simulink model "EcoSIM3_P2_C2"  (R2014b)
settings: Solver=ode1  SolverMode=SingleTasking  StartTime=0.0  StopTime=inf  FixedStep=0.01  RelTol=1e-3
PostLoadFcn:
  | %, if any(exist('dsrtsu_mdlpostloadfcn', 'file') == [2, 3, 6]), try dsrtsu_mdlpostloadfcn('Execute', bdroot); catch fprintf('Error in PostLoadFcn (dsrtsu_mdlpostloadfcn) for model "%s":\n %s\n', bdroot, lasterr); end, end,
InitFcn:
  | tic
  | %Startup_EcoSIM
undefined symbols (not defined in the file or in its folder): canChannel, Controls, DriveCycles, Driver, EM_EFF_MAP, EM_PwrLoss_MAP, EngPwr, EngSpd, EngTrq, Glbl, Plants, Power, Torque, Veh_Dynamics
libraries: canmsglib x100, canlib x87, fl_lib x78, simulink x59, nesl_utility x40, sdl_lib x17, dspsigops x5, dspswit3 x3, dspstat3 x2, commnoisgen2 x1, dspfdesign x1
(part 4 of 15)

== system EcoSIM3_P2_C2/Powertrain/Accessories/The Corrupter/Switch Logic1 ==
  F : Inport
  L : Inport  Port=2
  NF : Inport  Port=3
  Switch : Switch  Criteria=u2 ~= 0
  Out1 : Outport
  wires:
  L/1 -> Switch/2
  Switch/1 -> Out1/1
  NF/1 -> Switch/3
  F/1 -> Switch/1

== system EcoSIM3_P2_C2/Powertrain/BAS Motor/ Compnent Model/Actuators ==
  note: Actuator Model or a Signal Pass-through, Remove the bus if you are passing through all the signals
  ActuatorInputs : Inport
  Actuator Outputs : Outport
  wires:
  ActuatorInputs/1 -> Actuator Outputs/1

== system EcoSIM3_P2_C2/Powertrain/BAS Motor/ Compnent Model/Plant ==
  note: Component Level Performance Maps
  note: Three kinds of Outputs:
      | 1.To_sensors: Signals that can actually be sensed through Sensors go to sensor models
      | 2. To_plants: Signals that are not actually sensed by sensors but are utilized by the rest of the plant and actually happen physically
      | Component_Logging: Logs both the signal kinds before going through sensor
  note: Motor Speed
  From_Actuators : Inport
  Sensor_Feedback : Inport  Port=2
  BAS Max Torque Curve : Lookup  InputValues=Plants.BAS.Mdl.Plant.max_min_w  Table=Plants.BAS.Mdl.Plant.T_max_Peak  LookUpMeth=Interpolation-Use End Values  SaturateOnIntegerOverflow=on
  BAS Min Torque Curve : Lookup  InputValues=Plants.BAS.Mdl.Plant.max_min_w  Table=Plants.BAS.Mdl.Plant.T_min_Peak  LookUpMeth=Interpolation-Use End Values  SaturateOnIntegerOverflow=on
  Bus Selector : BusSelector  OutputSignals=BAS_Torque_Command_Nm
  Bus Selector1 : BusSelector  OutputSignals=BAS_Speed_rad_per_s
  Ideal Torque Source : fl_lib/Mechanical/Mechanical Sources/Ideal Torque Source
  Inertia : fl_lib/Mechanical/Rotational Elements/Inertia  inertia=0.02 kg*m^2  w_specify=off  w_priority=High  w=0 rad/s  t_specify=off  t_priority=High  t=0 N*m
  Mechanical Rotational Reference : fl_lib/Mechanical/Rotational Elements/Mechanical Rotational Reference
  Saturation Dynamic1 : simulink/Discontinuities/Saturation Dynamic  OutMin=[]  OutMax=[]  OutDataTypeStr=Inherit: Same as second input  OutDataType=sfix(16)  OutScaling=2^-10  DoSatur=off
  Simulink-PS Converter : nesl_utility/Simulink-PS Converter  PhysicalDomain=network_engine_domain  SubClassName=ps_input  LeftPortType=input  RightPortType=output  PseudoPeriodic=off  Frequencies=[]  NoiseDistribution=none  NoiseParameters=[]  Unit=N*m  AffineConversion=off  InputFiltering=off  SimscapeFilterOrder=1  InputFilterTimeConstant=0.001  UdotUserProvided=1
  To_Sensors : PMIOPort  Port=1  Side=Right
  wires:
  From_Actuators/1 -> Bus Selector/1
  BAS Max Torque Curve/1 -> Saturation Dynamic1/1
  BAS Min Torque Curve/1 -> Saturation Dynamic1/3
  Bus Selector/1 -> Saturation Dynamic1/2  "<BAS_Torque_Command_Nm>"
  Saturation Dynamic1/1 -> Simulink-PS Converter/1  "BAS_Torque_Out_Nm"
  Bus Selector1/1 -> BAS Min Torque Curve/1, BAS Max Torque Curve/1  "<BAS_Speed_rad_per_s>"
  Sensor_Feedback/1 -> Bus Selector1/1
  connections:
  Mechanical Rotational Reference/LConn1 -- Ideal Torque Source/RConn2
  Ideal Torque Source/RConn1 -- Simulink-PS Converter/RConn1
  Ideal Torque Source/LConn1 -- Inertia/LConn1 -- To_Sensors/RConn1

== system EcoSIM3_P2_C2/Powertrain/BAS Motor/ Compnent Model/Sensors ==
  note: Sensor Model: Place where we add Corrupter
  Bus Creator : BusCreator  Inputs=3
  Ideal Rotational Motion Sensor : fl_lib/Mechanical/Mechanical Sensors/Ideal Rotational Motion Sensor  offset=0 rad
  Ideal Torque Sensor : fl_lib/Mechanical/Mechanical Sensors/Ideal Torque Sensor
  Mechanical Rotational Reference1 : fl_lib/Mechanical/Rotational Elements/Mechanical Rotational Reference
  PS-Simulink Converter : nesl_utility/PS-Simulink Converter  PhysicalDomain=network_engine_domain  SubClassName=ps_output  LeftPortType=input  RightPortType=output  PseudoPeriodic=off  Frequencies=[]  Unit=rad/s  AffineConversion=off
  PS-Simulink Converter1 : nesl_utility/PS-Simulink Converter  PhysicalDomain=network_engine_domain  SubClassName=ps_output  LeftPortType=input  RightPortType=output  PseudoPeriodic=off  Frequencies=[]  Unit=N*m  AffineConversion=off
  Product : Product
  Sensor lag : Subsystem
  Sensor lag1 : Subsystem
  Shaft : PMIOPort  Port=1  Side=Left
  To_Belt : PMIOPort  Port=2  Side=Right
  Sensor Out : Outport
  Battery : Outport  Port=2
  wires:
  Bus Creator/1 -> Sensor Out/1  "BAS_Sensor_Out"
  Sensor lag/1(o) -> Product/1, Bus Creator/1  "BAS_Speed_rad_per_s"
  PS-Simulink Converter1/1 -> Sensor lag1/1(i)  "BAS_Torque_Out_Nm"
  Product/1 -> Battery/1, Bus Creator/3  "BAS_Power_Out_W"
  PS-Simulink Converter/1 -> Sensor lag/1(i)  "BAS_Speed_rad_per_s"
  Sensor lag1/1(o) -> Product/2, Bus Creator/2  "BAS_Torque_Out_Nm"
  connections:
  Shaft/RConn1 -- Ideal Rotational Motion Sensor/LConn1 -- Ideal Torque Sensor/LConn1
  Ideal Rotational Motion Sensor/RConn1 -- Mechanical Rotational Reference1/LConn1
  PS-Simulink Converter1/LConn1 -- Ideal Torque Sensor/RConn2
  PS-Simulink Converter/LConn1 -- Ideal Rotational Motion Sensor/RConn2
  To_Belt/RConn1 -- Ideal Torque Sensor/RConn1

== system EcoSIM3_P2_C2/Powertrain/BAS Motor/Soft ECU/Algorithm ==
  note: Does ModeRequest require a handshake from the super?
      | There is no Lockout. Right now, Super sends mode request
      | 1 constantly
  note: Signals like T& E are used to calculate whatever is required by Soft ECU
  note: Sensor signals getting transmitted over CAN are selected here
  note: Signals getting transmitted to Actuators are bussed together here
  note: Signals getting transmitted to Actuators are bussed together here
  Inputs : Inport
  BAS_Stateflow : Subsystem
  Bus Creator3 : BusCreator  Inputs=8
  Bus Selector : BusSelector  OutputSignals=BAS_Sensor_Out,BAS_SoftECU_Receive.BAS_CAN.SetValues.BAS_Mode_Request,BAS_SoftECU_Receive.BAS_CAN.SetValues.BAS_Torque_Request_Nm,BAS_SoftECU_Receive.BAS_Electrical.BAS_Powerup
  Bus Selector1 : BusSelector  OutputSignals=BAS_Speed_rad_per_s,BAS_Torque_Out_Nm
  Bus Selector2 : BusSelector  Commented=on  OutputSignals=BAS_Powerup
  Bus Selector3 : BusSelector  OutputSignals=BAS_Status_Mode,BAS_Fault_Status,Fault_U,Fault_V,Fault_W
  Constant : Constant  Value=60
  Display : Display
  Display1 : Display
  For_testing : Constant  Value=2250  SampleTime=0.01
  From : From  Commented=on  GotoTag=Powerups  TagVisibility=global
  Outputs : Outport
  wires:
  Inputs/1 -> Bus Selector/1
  Bus Selector/1 -> Bus Selector1/1  "<BAS_Sensor_Out>"
  Bus Selector1/1 -> Bus Creator3/2, BAS_Stateflow/4(MotorSpeed)  "<BAS_Speed_rad_per_s>"
  Bus Creator3/1 -> Outputs/1  "BAS_CAN_Out"
  BAS_Stateflow/1(BAS_Torque_Command_Nm) -> Bus Creator3/3, Display/1  "BAS_Torque_Command_Nm"
  BAS_Stateflow/2(BAS_CAN_Out) -> Bus Selector3/1
  Bus Selector3/1 -> Bus Creator3/4  "<BAS_Status_Mode>"
  Bus Selector3/3 -> Bus Creator3/6  "<Fault_U>"
  Bus Selector3/4 -> Bus Creator3/7  "<Fault_V>"
  Bus Selector3/5 -> Bus Creator3/8  "<Fault_W>"
  Constant/1 -> BAS_Stateflow/2(TorqueLimit)
  Bus Selector/2 -> BAS_Stateflow/1(ModeRequest)  "<BAS_Mode_Request>"
  Bus Selector/3 -> BAS_Stateflow/3(TorqueCommand), Display1/1  "<BAS_Torque_Request_Nm>"
  Bus Selector3/2 -> Bus Creator3/5  "<BAS_Fault_Status>"
  From/1 -> Bus Selector2/1
  Bus Selector/4 -> BAS_Stateflow/5(PowerUp)  "<BAS_Powerup>"
  For_testing/1 -> BAS_Stateflow/6(Speed_cmd)
  Bus Selector1/2 -> Bus Creator3/1  "<BAS_Torque_Out_Nm>"

== system EcoSIM3_P2_C2/Powertrain/BAS Motor/Soft ECU/Inputs ==
  note: Do the input conditioning (if any) required by the
      | Algorith
  note: Select the CAN signals
  note: Select the Sensor signals
  note: Combine all the Signals that go to the
      | Soft ECU Algorithm:
      | -Calculated Signals from Sensors and CAN
      | -Signalfrom sensors pass through because they
      | need to be sent out over the CAN by the ECU
  CAN_In : Inport
  Sensors : Inport  Port=2
  Bus Creator : BusCreator  Inputs=3
  Bus Selector1 : BusSelector  OutputSignals=BAS_Speed_rad_per_s
  To_Algorithm : Outport
  wires:
  Sensors/1 -> Bus Creator/1, Bus Selector1/1  "BAS_Sensor_Out"
  Bus Creator/1 -> To_Algorithm/1  "Component_to_Alg"
  Bus Selector1/1 -> Bus Creator/2  "<BAS_Speed_rad_per_s>"
  CAN_In/1 -> Bus Creator/3

== system EcoSIM3_P2_C2/Powertrain/BAS Motor/Soft ECU/Inputs1 ==
  From Algorithm : Inport
  Bus Creator1 : BusCreator  Inputs=2
  Bus Creator3 : BusCreator  Inputs=8
  Bus Selector : BusSelector  OutputSignals=BAS_Speed_rad_per_s,BAS_Torque_Command_Nm,BAS_Status_Mode,BAS_Torque_Out_Nm,BAS_Fault_Status,Fault_U,Fault_V,Fault_W
  CAN Out : Outport
  Actuator Cmds : Outport  Port=2
  wires:
  From Algorithm/1 -> Bus Selector/1
  Bus Creator1/1 -> Actuator Cmds/1  "BAS_Actuator_Cmds"
  Bus Creator3/1 -> CAN Out/1  "BAS_CAN_Out"
  Bus Selector/1 -> Bus Creator3/1, Bus Creator1/1  "<BAS_Speed_rad_per_s>"
  Bus Selector/2 -> Bus Creator3/2, Bus Creator1/2  "<BAS_Torque_Command_Nm>"
  Bus Selector/3 -> Bus Creator3/3  "<BAS_Status_Mode>"
  Bus Selector/8 -> Bus Creator3/7  "<Fault_W>"
  Bus Selector/7 -> Bus Creator3/6  "<Fault_V>"
  Bus Selector/6 -> Bus Creator3/5  "<Fault_U>"
  Bus Selector/5 -> Bus Creator3/4  "<BAS_Fault_Status>"
  Bus Selector/4 -> Bus Creator3/8  "<BAS_Torque_Out_Nm>"

== system EcoSIM3_P2_C2/Powertrain/Charger/Soft ECU/Algorithm ==
  note: Both outputs are digital signals
  note: Signals like T& E are used to calculate whatever is required by Soft ECU
  Inputs : Inport
  Brusa SoftECU : Stateflow chart  TreatAsAtomicUnit=on
  Bus Creator1 : BusCreator  Inputs=3
  Bus Selector : BusSelector  OutputSignals=AC_Supply,PON
  Outputs : Outport
  wires:
  Bus Creator1/1 -> Outputs/1  "Brusa_SoftECU_Out"
  Inputs/1 -> Bus Selector/1
  Bus Selector/1 -> Brusa SoftECU/1(AC_Supply)  "<AC_Supply>"
  Bus Selector/2 -> Brusa SoftECU/2(PON)  "<PON>"
  Brusa SoftECU/1(chga_wake) -> Bus Creator1/1
  Brusa SoftECU/2(GCM_Wakeup_charge) -> Bus Creator1/2
  Brusa SoftECU/3(charge_start) -> Bus Creator1/3

== system EcoSIM3_P2_C2/Powertrain/Charger/Soft ECU/Inputs ==
  note: Combine all the Signals that go to the
      | Soft ECU Algorithm:
      | -Calculated Signals from Sensors and CAN
      | -Signalfrom sensors pass through because they
      | need to be sent out over the CAN by the ECU
  note: Select the Sensor signals
  note: Select the CAN signals
  FromESS1 : Inport
  Supply : Inport  Port=2
  Bus Creator : BusCreator  Inputs=2
  To_Algorithm : Outport
  wires:
  Supply/1 -> Bus Creator/2  "AC_Supply"
  Bus Creator/1 -> To_Algorithm/1  "Inputs"
  FromESS1/1 -> Bus Creator/1

== system EcoSIM3_P2_C2/Powertrain/Charger/Soft ECU/Outputs ==
  note: Select the Sensor signals
  From Algorithm : Inport
  Bus Creator : BusCreator  Inputs=2
  Bus Creator1 : BusCreator  Inputs=1
  Bus Selector : BusSelector  OutputSignals=chga_wake,GCM_Wakeup_charge,charge_start
  ToECUs : Outport
  Actuator_Cmds : Outport  Port=2
  wires:
  From Algorithm/1 -> Bus Selector/1
  Bus Selector/1 -> Bus Creator/1  "<chga_wake>"
  Bus Selector/2 -> Bus Creator/2  "<GCM_Wakeup_charge>"
  Bus Creator/1 -> ToECUs/1  "Brusa_Out"
  Bus Selector/3 -> Bus Creator1/1  "<charge_start>"
  Bus Creator1/1 -> Actuator_Cmds/1  "Actuator_Cmds"

== system EcoSIM3_P2_C2/Powertrain/Clutch_Transmission2/CP1 SoftEcu/Algorithm ==
  note: Cignals getting transmitted to Actuators are bussed together here
  note: Sensor signals getting transmitted over CAN are bussed together here
  note: Sensor signals getting transmitted over CAN are selected here
  note: Signals like T& E are used to calculate whatever is required by Soft ECU
  Inputs : Inport
  Bus Creator : BusCreator  Inputs=2
  Bus Creator1 : BusCreator  Inputs=1
  Bus Creator2 : BusCreator  Inputs=1
  Bus Selector : BusSelector  OutputSignals=Clutch_Request,Sensor_Out.Clutch_Sensor_Out.Clutch_Pressure
  Chart : Stateflow chart  TreatAsAtomicUnit=on
  Memory : Memory  X0=120
  Outputs : Outport
  wires:
  Inputs/1 -> Bus Selector/1
  Chart/1(Clutch_Engage) -> Bus Creator1/1  "Clutch_Engage"
  Bus Creator1/1 -> Bus Creator/1  "Component_Actuator_Commands"
  Bus Creator2/1 -> Bus Creator/2  "Clutch_CAN_Out"
  Bus Selector/2 -> Memory/1  "<Clutch_Pressure>"
  Chart/2(Clutch_Sw) -> Bus Creator2/1  "Clutch_Sw"
  Bus Selector/1 -> Chart/1(Clutch_Request)  "<Clutch_Request>"
  Memory/1 -> Chart/2(Clutch_Pressure)
  Bus Creator/1 -> Outputs/1

== system EcoSIM3_P2_C2/Powertrain/Clutch_Transmission2/CP1 SoftEcu/Inputs ==
  note: Combine all the Signals that go to the
      | Soft ECU Algorithm:
      | -Calculated Signals from Sensors and CAN
      | -Signalfrom sensors pass through because they
      | need to be sent out over the CAN by the ECU
  note: Select the Sensor signals
  note: Select the CAN signals
  note: Do the input conditioning (if any) required by the
      | Algorith
  Sensors : Inport
  From GCM : Inport  Port=2
  Bus Creator : BusCreator  Inputs=2
  Bus Selector : BusSelector  OutputSignals=Clutch_Request
  To_Algorithm : Outport
  wires:
  Bus Creator/1 -> To_Algorithm/1  "Component_to_Alg"
  Sensors/1 -> Bus Creator/1  "Sensor_Out"
  From GCM/1 -> Bus Selector/1
  Bus Selector/1 -> Bus Creator/2  "<Clutch_Request>"

== system EcoSIM3_P2_C2/Powertrain/Clutch_Transmission2/CP1 SoftEcu/Inputs1 ==
  From Algorithm : Inport
  Bus Selector : BusSelector  OutputSignals=Component_Actuator_Commands.Clutch_Engage,Clutch_CAN_Out
  Actuator Cmd : Outport
  To GCM : Outport  Port=2
  wires:
  From Algorithm/1 -> Bus Selector/1  "Sensor_Out"
  Bus Selector/1 -> Actuator Cmd/1  "<Clutch_Engage>"
  Bus Selector/2 -> To GCM/1  "<Clutch_CAN_Out>"

== system EcoSIM3_P2_C2/Powertrain/Clutch_Transmission2/Clutch_Plant/Custom Clutch ==
  -1 : fl_lib/Physical Signals/Functions/PS Gain  gain=-1
  Dynamic friction coefficient lookup table : fl_lib/Physical Signals/Lookup Tables/PS Lookup Table (1D)  x_t=[ 0 0.1 0.2 0.3 0.4 0.5 1 2 5 10 100 1000 ]  y_t=[ 0.29 0.28 0.26 0.22 0.21 0.2 0.2 0.19 0.19 0.19 0.19 0.19 ]  interp_method=1  extrap_method=1
  Effective radius : fl_lib/Physical Signals/Functions/PS Gain  gain=0.3
  Fundamental Friction Clutch : sdl_lib/Clutches/Fundamental Components/Fundamental Friction Clutch  unidirectional=0  w_tol=0.001 rad/s  initial_state_locked=0
  PS Abs : fl_lib/Physical Signals/Nonlinear Operators/PS Abs
  PS Product1 : fl_lib/Physical Signals/Functions/PS Product
  PS-Simulink Converter1 : nesl_utility/PS-Simulink Converter  PhysicalDomain=network_engine_domain  SubClassName=ps_output  LeftPortType=input  RightPortType=output  PseudoPeriodic=off  Frequencies=[]  Unit=rad/s  AffineConversion=off
  Peak force : fl_lib/Physical Signals/Functions/PS Gain  gain=10
  Slip(rad/s) : Scope
      settings: YMin=-4  YMax=1
  Static/dynamic friction ratio : fl_lib/Physical Signals/Functions/PS Gain  gain=1.1
  "[0, inf]" : fl_lib/Physical Signals/Nonlinear Operators/PS Saturation  upper_limit=inf  lower_limit=0
  P : PMIOPort  Port=1  Side=Left
  Mode : PMIOPort  Port=2  Side=Right
  F : PMIOPort  Port=3  Side=Right
  B : PMIOPort  Port=4  Side=Left
  wires:
  PS-Simulink Converter1/1 -> Slip(rad/s)/1
  connections:
  Peak force/RConn1 -- PS Product1/LConn1
  PS Product1/RConn1 -- Effective radius/LConn1
  "[0, inf]"/RConn1 -- Peak force/LConn1
  Fundamental Friction Clutch/RConn3 -- F/RConn1
  Fundamental Friction Clutch/RConn2 -- Mode/RConn1
  PS-Simulink Converter1/LConn1 -- Fundamental Friction Clutch/RConn1 -- PS Abs/LConn1
  B/RConn1 -- Fundamental Friction Clutch/LConn4
  P/RConn1 -- "[0, inf]"/LConn1
  Fundamental Friction Clutch/LConn2 -- -1/LConn1 -- Static/dynamic friction ratio/RConn1
  Effective radius/RConn1 -- Fundamental Friction Clutch/LConn1 -- Static/dynamic friction ratio/LConn1
  Dynamic friction coefficient lookup table/RConn1 -- PS Product1/LConn2
  -1/RConn1 -- Fundamental Friction Clutch/LConn3
  PS Abs/RConn1 -- Dynamic friction coefficient lookup table/LConn1

== system EcoSIM3_P2_C2/Powertrain/Clutch_Transmission2/Clutch_Plant/Sensors ==
  Clutch_Pressure : Inport
  Bus Creator : BusCreator  Inputs=1
  Ideal Rotational Motion Sensor : fl_lib/Mechanical/Mechanical Sensors/Ideal Rotational Motion Sensor  offset=0 rad
  Ideal Torque Sensor : fl_lib/Mechanical/Mechanical Sensors/Ideal Torque Sensor
  Mechanical Rotational Reference1 : fl_lib/Mechanical/Rotational Elements/Mechanical Rotational Reference
  PS-Simulink Converter : nesl_utility/PS-Simulink Converter  PhysicalDomain=network_engine_domain  SubClassName=ps_output  LeftPortType=input  RightPortType=output  PseudoPeriodic=off  Frequencies=[]  Unit=rad/s  AffineConversion=off
  PS-Simulink Converter1 : nesl_utility/PS-Simulink Converter  PhysicalDomain=network_engine_domain  SubClassName=ps_output  LeftPortType=input  RightPortType=output  PseudoPeriodic=off  Frequencies=[]  Unit=N*m  AffineConversion=off
  Terminator : Terminator
  Terminator1 : Terminator
  Shaft : PMIOPort  Port=1  Side=Left
  To_Trans : PMIOPort  Tag=PMCPort  Port=2  Side=Right
  Clutch_Status : Outport
  wires:
  PS-Simulink Converter/1 -> Terminator/1  "Clutch_Speed_rad_per_s"
  PS-Simulink Converter1/1 -> Terminator1/1  "Clutch_Torque_Out_Nm"
  Clutch_Pressure/1 -> Bus Creator/1  "Clutch_Pressure"
  Bus Creator/1 -> Clutch_Status/1  "Clutch_Sensor_Out"
  connections:
  Ideal Torque Sensor/LConn1 -- Shaft/RConn1 -- Ideal Rotational Motion Sensor/LConn1
  Ideal Rotational Motion Sensor/RConn1 -- Mechanical Rotational Reference1/LConn1
  PS-Simulink Converter/LConn1 -- Ideal Rotational Motion Sensor/RConn2
  PS-Simulink Converter1/LConn1 -- Ideal Torque Sensor/RConn2
  To_Trans/RConn1 -- Ideal Torque Sensor/RConn1

== system EcoSIM3_P2_C2/Powertrain/Clutch_Transmission2/GCM/GCM Soft ECU ==
  Inputs : Inport
  Bus Creator : BusCreator
  Bus Selector : BusSelector  OutputSignals=Trans_Receive.Gear_Request,SoftECU_Out.Trans_CAN_Out.Actual_Gear
  Display : Display
  Display1 : Display
  Memory : Memory
  Shift Signal Generator : Stateflow chart  TreatAsAtomicUnit=on
  Outputs : Outport
  wires:
  Shift Signal Generator/1(Clutch_Request) -> Bus Creator/1  "Clutch_Request"
  Inputs/1 -> Bus Selector/1
  Shift Signal Generator/2(Upshift_Sw) -> Bus Creator/2  "Upshift_Sw"
  Shift Signal Generator/3(Downshift_Sw) -> Bus Creator/3  "Downshift_Sw"
  Bus Selector/1 -> Display/1, Shift Signal Generator/1(Gear_Request)  "<Gear_Request>"
  Bus Selector/2 -> Memory/1  "<Actual_Gear>"
  Bus Creator/1 -> Outputs/1
  Memory/1 -> Display1/1, Bus Creator/4, Shift Signal Generator/2(Actual_Gear)  "Actual_Gear"

== system EcoSIM3_P2_C2/Powertrain/Clutch_Transmission2/GCM/Inputs ==
  note: Do the input conditioning (if any) required by the
      | Algorith
  note: Select the CAN signals
  note: Select the Sensor signals
  note: Combine all the Signals that go to the
      | Soft ECU Algorithm:
      | -Calculated Signals from Sensors and CAN
      | -Signalfrom sensors pass through because they
      | need to be sent out over the CAN by the ECU
  From SoftECU : Inport
  CAN_In : Inport  Port=2
  Bus Creator : BusCreator  Inputs=2
  Bus Selector : BusSelector  OutputSignals=Clutch_Trans_SoftECU_Receive.Clutch_Trans_CAN.Trans_Receive
  To_Algorithm : Outport
  wires:
  CAN_In/1 -> Bus Selector/1
  From SoftECU/1 -> Bus Creator/1
  Bus Creator/1 -> To_Algorithm/1  "Component_to_Alg"
  Bus Selector/1 -> Bus Creator/2  "<Trans_Receive>"

== system EcoSIM3_P2_C2/Powertrain/Clutch_Transmission2/GCM/Outputs ==
  From Algorithm : Inport
  Bus Creator : BusCreator  Inputs=3
  Bus Creator1 : BusCreator  Inputs=1
  Bus Selector : BusSelector  OutputSignals=Actual_Gear,Clutch_Request,Upshift_Sw,Downshift_Sw
  CAN_Out : Outport
  To_SoftECU : Outport  Port=2
  wires:
  From Algorithm/1 -> Bus Selector/1  "Sensor_Out"
  Bus Selector/2 -> Bus Creator/1  "<Clutch_Request>"
  Bus Selector/3 -> Bus Creator/2  "<Upshift_Sw>"
  Bus Selector/4 -> Bus Creator/3  "<Downshift_Sw>"
  Bus Creator/1 -> To_SoftECU/1  "SoftECU_Receive"
  Bus Creator1/1 -> CAN_Out/1  "Message_1"
  Bus Selector/1 -> Bus Creator1/1  "<Actual_Gear>"

== system EcoSIM3_P2_C2/Powertrain/Clutch_Transmission2/Mastershift Softecu/Algorithm ==
  note: Signals like T& E are used to calculate whatever is required by Soft ECU
  note: Sensor signals getting transmitted over CAN are selected here
  note: Cignals getting transmitted to Actuators are bussed together here
  Inputs : Inport
  Add4 : Sum
  Bus Creator : BusCreator  Inputs=2
  Bus Selector : BusSelector  OutputSignals=Clutch_Sw,Sensor_Out.Trans_Sensor_Out.Actual_Gear,Upshift_Sw,Downshift_Sw
  Chart : Stateflow chart  TreatAsAtomicUnit=on
  Display : Display
  Display1 : Display
  Downshift Counter : dspswit3/Counter  Direction=Up  CountEvent=Rising edge  CounterSize=User defined  MaxCount=255  InitialCount=0  Output=Count  HitValue=32  ResetInput=on  SamplesPerFrame=1  Ts=1  CntDtype=double  HitDtype=Logical
  Gain : Gain  Gain=-1
  Memory : Memory
  Memory1 : Memory
  Upshift Counter : dspswit3/Counter  Direction=Up  CountEvent=Rising edge  CounterSize=User defined  MaxCount=255  InitialCount=0  Output=Count  HitValue=32  ResetInput=on  SamplesPerFrame=1  Ts=1  CntDtype=double  HitDtype=Logical
  Outputs : Outport
  wires:
  Inputs/1 -> Bus Selector/1
  Bus Selector/2 -> Memory/1  "<Actual_Gear>"
  Bus Selector/1 -> Chart/1(Clutch_Sw)  "<Clutch_Sw>"
  Chart/2(TCM_Gear) -> Bus Creator/2  "TCM_Gear"
  Upshift Counter/1 -> Add4/1
  Downshift Counter/1 -> Gain/1
  Gain/1 -> Add4/2
  Bus Selector/3 -> Upshift Counter/1  "<Upshift_Sw>"
  Bus Selector/4 -> Downshift Counter/1  "<Downshift_Sw>"
  Add4/1 -> Chart/3(Count), Display1/1
  Chart/3(reset) -> Memory1/1  "reset"
  Memory/1 -> Chart/2(Actual_Gear)
  Bus Creator/1 -> Outputs/1
  Memory1/1 -> Downshift Counter/2, Upshift Counter/2
  Chart/1(Gear_Cmd) -> Display/1, Bus Creator/1

== system EcoSIM3_P2_C2/Powertrain/Clutch_Transmission2/Mastershift Softecu/Inputs ==
  note: Do the input conditioning (if any) required by the
      | Algorith
  note: Select the CAN signals
  note: Select the Sensor signals
  note: Combine all the Signals that go to the
      | Soft ECU Algorithm:
      | -Calculated Signals from Sensors and CAN
      | -Signalfrom sensors pass through because they
      | need to be sent out over the CAN by the ECU
  Sensors : Inport
  From GCM : Inport  Port=2
  Clutch_CAN_Out : Inport  Port=3
  Bus Creator : BusCreator
  Bus Selector : BusSelector  OutputSignals=Upshift_Sw,Downshift_Sw
  Bus Selector1 : BusSelector  OutputSignals=Clutch_Sw
  To_Algorithm : Outport
  wires:
  From GCM/1 -> Bus Selector/1
  Sensors/1 -> Bus Creator/1
  Bus Creator/1 -> To_Algorithm/1  "Component_to_Alg"
  Clutch_CAN_Out/1 -> Bus Selector1/1
  Bus Selector1/1 -> Bus Creator/4  "<Clutch_Sw>"
  Bus Selector/1 -> Bus Creator/2  "<Upshift_Sw>"
  Bus Selector/2 -> Bus Creator/3  "<Downshift_Sw>"

== system EcoSIM3_P2_C2/Powertrain/Clutch_Transmission2/Mastershift Softecu/Outputs ==
  note: Combine all the Signals that go to the
      | Soft ECU Algorithm:
      | -Calculated Signals from Sensors and CAN
      | -Signalfrom sensors pass through because they
      | need to be sent out over the CAN by the ECU
  From Algorithm : Inport
  Bus Creator : BusCreator  Inputs=1
  Bus Selector : BusSelector  OutputSignals=Gear_Cmd,TCM_Gear
  Actuator Commands : Outport
  To GCM : Outport  Port=2
  wires:
  From Algorithm/1 -> Bus Selector/1
  Bus Selector/1 -> Bus Creator/1  "<Gear_Cmd>"
  Bus Selector/2 -> To GCM/1  "<TCM_Gear>"
  Bus Creator/1 -> Actuator Commands/1  "Trans_Actuator_Commands"

== system EcoSIM3_P2_C2/Powertrain/Clutch_Transmission2/Trans_Plant/Actuators ==
  note: Actuator Model or a Signal Pass-through, Remove the bus if you are passing through all the signals
  ActuatorInputs : Inport
  Actuator Outputs : Outport
  wires:
  ActuatorInputs/1 -> Actuator Outputs/1

== system EcoSIM3_P2_C2/Powertrain/Clutch_Transmission2/Trans_Plant/Plant ==
  note: Try to detect actual gears from simscape model. Using reverse lookup from rate limiter starts giving value from Gear 5, because it has the lowest ratio
  note: Component Level Performance Maps
  From_Actuators : Inport
  Bus Selector : BusSelector  OutputSignals=Clutch_Trans_SoftECU_Receive.Clutch_Trans_CAN.Trans_Receive.Gear_Request
  Input Shaft Inertia : fl_lib/Mechanical/Rotational Elements/Inertia  inertia=0.01 kg*m^2  w_specify=off  w_priority=High  w=580*2*pi/60 rad/s  t_specify=off  t_priority=High  t=0 N*m
  Output Shaft Inertia1 : fl_lib/Mechanical/Rotational Elements/Inertia  inertia=.01 kg*m^2  w_specify=off  w_priority=High  w=580*2*pi/60 rad/s  t_specify=off  t_priority=High  t=0 N*m
  Rate Limiter : RateLimiter  RisingSlewLimit=2  FallingSlewLimit=-2  SampleTimeMode=inherited  InitialCondition=2.95
  ReverseLookup : Lookup  InputValues=[0 0.6300 1 1.3400 1.9400 2.9500]  Table=[0 5 4 3 2 1]  LookUpMeth=Use Input Nearest
  Simulink-PS Converter : nesl_utility/Simulink-PS Converter  PhysicalDomain=network_engine_domain  SubClassName=ps_input  LeftPortType=input  RightPortType=output  PseudoPeriodic=off  Frequencies=[]  NoiseDistribution=none  NoiseParameters=[]  Unit=1  AffineConversion=off  InputFiltering=off  SimscapeFilterOrder=1  InputFilterTimeConstant=0.001  UdotUserProvided=1
  Trans GR : Lookup  InputValues=Plants.Trans.Mdl.Plant.Gear_cmd  Table=Plants.Trans.Mdl.Plant.GR  LookUpMeth=Use Input Nearest
  Variable Ratio Transmission : sdl_lib/Couplings & Drives/Variable Ratio Transmission  rotation_direction=1  kp=3e+5 N*m/rad  kv=0.05 N*m/(rad/s)  initial_torque=0 N*m  losses_model=1  efficiency=0.8  mu_visc=[ 0 0 ] N*m/(rad/s)  w_thr=0.01 rad/s
  Trans Input Shaft : PMIOPort  Port=1  Side=Left
  To Sensors : PMIOPort  Port=2  Side=Right
  Actual_Gear : Outport
  wires:
  Bus Selector/1 -> Trans GR/1  "<Gear_Request>"
  From_Actuators/1 -> Bus Selector/1
  ReverseLookup/1 -> Actual_Gear/1
  Trans GR/1 -> Rate Limiter/1
  Rate Limiter/1 -> ReverseLookup/1, Simulink-PS Converter/1
  connections:
  Trans Input Shaft/RConn1 -- Input Shaft Inertia/LConn1 -- Variable Ratio Transmission/LConn2
  Variable Ratio Transmission/RConn1 -- Output Shaft Inertia1/LConn1 -- To Sensors/RConn1
  Simulink-PS Converter/RConn1 -- Variable Ratio Transmission/LConn1

== system EcoSIM3_P2_C2/Powertrain/Clutch_Transmission2/Trans_Plant/Sensors ==
  note: Sensor Model: Place where we add Corrupter
  Actual_Gear : Inport
  Bus Creator : BusCreator  Inputs=3
  Ideal Rotational Motion Sensor : fl_lib/Mechanical/Mechanical Sensors/Ideal Rotational Motion Sensor  offset=0 rad
  Ideal Torque Sensor : fl_lib/Mechanical/Mechanical Sensors/Ideal Torque Sensor
  Mechanical Rotational Reference1 : fl_lib/Mechanical/Rotational Elements/Mechanical Rotational Reference
  PS-Simulink Converter : nesl_utility/PS-Simulink Converter  PhysicalDomain=network_engine_domain  SubClassName=ps_output  LeftPortType=input  RightPortType=output  PseudoPeriodic=off  Frequencies=[]  Unit=1  AffineConversion=off
  PS-Simulink Converter1 : nesl_utility/PS-Simulink Converter  PhysicalDomain=network_engine_domain  SubClassName=ps_output  LeftPortType=input  RightPortType=output  PseudoPeriodic=off  Frequencies=[]  Unit=N*m  AffineConversion=off
  Trans Output Shaft : PMIOPort  Port=1  Side=Left
  To_MC : PMIOPort  Tag=PMCPort  Port=2  Side=Right
  Sensor Out : Outport
  ActGear : Outport  Port=2
  wires:
  Bus Creator/1 -> Sensor Out/1  "Trans_Sensor"
  PS-Simulink Converter1/1 -> Bus Creator/3  "Trans_Torque_Out_Nm"
  PS-Simulink Converter/1 -> Bus Creator/2  "Trans_Speed_rad_per_s"
  Actual_Gear/1 -> ActGear/1, Bus Creator/1  "Actual_Gear"
  connections:
  To_MC/RConn1 -- Ideal Torque Sensor/RConn1
  PS-Simulink Converter/LConn1 -- Ideal Rotational Motion Sensor/RConn2
  PS-Simulink Converter1/LConn1 -- Ideal Torque Sensor/RConn2
  Ideal Rotational Motion Sensor/RConn1 -- Mechanical Rotational Reference1/LConn1
  Trans Output Shaft/RConn1 -- Ideal Rotational Motion Sensor/LConn1 -- Ideal Torque Sensor/LConn1

== system EcoSIM3_P2_C2/Powertrain/Electric Motor / Component Model/Actuators ==
  note: Actuator Model or a Signal Pass-through, Remove the bus if you are passing through all the signals
  ActuatorInputs : Inport
  Bus Creator : BusCreator  Inputs=1
  Bus Selector : BusSelector  OutputSignals=Commanded_Torque
  Gain : Gain
  Actuator Outputs : Outport
  wires:
  ActuatorInputs/1 -> Bus Selector/1
  Bus Selector/1 -> Gain/1  "<Commanded_Torque>"
  Gain/1 -> Bus Creator/1  "EM_Torque_Request_Nm"
  Bus Creator/1 -> Actuator Outputs/1

== system EcoSIM3_P2_C2/Powertrain/Electric Motor / Component Model/Plant ==
  note: Component Level Performance Maps
  note: Three kinds of Outputs:
      | 1.To_sensors: Signals that can actually be sensed through Sensors go to sensor models
      | 2. To_plants: Signals that are not actually sensed by sensors but are utilized by the rest of the plant and actually happen physically
      | Component_Logging: Logs both the signal kinds before going through sensor
  note: Component Level Performance Maps
  From_Actuators : Inport
  Sensor_Feedback : Inport  Port=2
  Bus Creator : BusCreator  Inputs=2
  Bus Selector : BusSelector  OutputSignals=EM_Torque_Request_Nm
  Bus Selector1 : BusSelector  OutputSignals=EM_Speed_produced_rad_per_s
  EM Efficiency : Lookup2D  Commented=on  RowIndex=Plants.EM.Mdl.Plant.w_rad  ColumnIndex=Plants.EM.Mdl.Plant.T_Nm  Table=Plants.EM.Mdl.Plant.Eff  LookUpMeth=Interpolation-Use End Values  SaturateOnIntegerOverflow=on  InputSameDT=on
  EM Max Torque Curve : Lookup  InputValues=Plants.EM.Mdl.Plant.max_min_w  Table=Plants.EM.Mdl.Plant.T_max_Peak  LookUpMeth=Interpolation-Use End Values  SaturateOnIntegerOverflow=on
  EM Min Torque Curve : Lookup  InputValues=Plants.EM.Mdl.Plant.max_min_w  Table=Plants.EM.Mdl.Plant.T_min_Peak  LookUpMeth=Interpolation-Use End Values  SaturateOnIntegerOverflow=on
  EM Power Loss : Lookup2D  RowIndex=Plants.EM.Mdl.Plant.w_rad_PL  ColumnIndex=Plants.EM.Mdl.Plant.T_Nm_PL  Table=Plants.EM.Mdl.Plant.power_loss  LookUpMeth=Interpolation-Use End Values  SaturateOnIntegerOverflow=on  InputSameDT=on
  EM_Thermal_Model : Subsystem
  Ideal Torque Source1 : fl_lib/Mechanical/Mechanical Sources/Ideal Torque Source
  Inertia1 : fl_lib/Mechanical/Rotational Elements/Inertia  inertia=0.2 kg*m^2  w_specify=off  w_priority=High  w=0 rad/s  t_specify=off  t_priority=High  t=0 N*m
  InternalMotorError : Constant  Value=0
  Mechanical Rotational Reference1 : fl_lib/Mechanical/Rotational Elements/Mechanical Rotational Reference
  Saturation Dynamic1 : simulink/Discontinuities/Saturation Dynamic  OutMin=[]  OutMax=[]  OutDataTypeStr=Inherit: Same as second input  OutDataType=sfix(16)  OutScaling=2^-10  DoSatur=off
  Simulink-PS Converter1 : nesl_utility/Simulink-PS Converter  PhysicalDomain=network_engine_domain  SubClassName=ps_input  LeftPortType=input  RightPortType=output  PseudoPeriodic=off  Frequencies=[]  NoiseDistribution=none  NoiseParameters=[]  Unit=N*m  AffineConversion=off  InputFiltering=off  SimscapeFilterOrder=1  InputFilterTimeConstant=.001  UdotUserProvided=1
  Solver Configuration1 : nesl_utility/Solver Configuration  PhysicalDomain=network_engine_domain  SubClassName=solver  LeftPortType=input  RightPortType=generic  Accelerate=off  Tones=[]  Harmonics=[]  SimulateNoise=off  Profile=off  UseLocalSampling=off  EnableSwitchedLinearOptims=on  FrequencyDomain=off  UseCCode=off  RelTol=0.001  AbsTol=1e-06  MinStep=1e-09  ToWorkspace=off  DoDC=off  ResidualTolerance=1e-9  UseLocalSolver=on  LocalSolverChoice=NE_BACKWARD_EULER_ADVANCER  LocalSolverSampleTime=.01  DoFixedCost=off  MaxNonlinIter=3  MaxModeIter=2  LinearAlgebra=Sparse  DelaysMemoryBudget=1024  AutomaticFiltering=on  FilteringTimeConstant=0.001
  To_Plants1 : PMIOPort  Port=1  Side=Right
  To_Sensors : Outport
  wires:
  Bus Creator/1 -> To_Sensors/1  "EM_to_sensors"
  From_Actuators/1 -> Bus Selector/1
  EM Max Torque Curve/1 -> Saturation Dynamic1/1
  EM Min Torque Curve/1 -> Saturation Dynamic1/3
  Bus Selector/1 -> Saturation Dynamic1/2  "<EM_Torque_Request_Nm>"
  InternalMotorError/1 -> Bus Creator/1  "InternalMotorError"
  Sensor_Feedback/1 -> Bus Selector1/1
  Bus Selector1/1 -> EM Power Loss/1, EM Min Torque Curve/1, EM Max Torque Curve/1  "<EM_Speed_produced_rad_per_s>"
  Saturation Dynamic1/1 -> EM Power Loss/2, Simulink-PS Converter1/1
  EM Power Loss/1 -> EM_Thermal_Model/1(EM_Power_Loss)  "EM_Power_Loss"
  EM_Thermal_Model/1(Out1) -> Bus Creator/2
  connections:
  Simulink-PS Converter1/RConn1 -- Ideal Torque Source1/RConn1
  Ideal Torque Source1/LConn1 -- To_Plants1/RConn1 -- Inertia1/LConn1 -- Solver Configuration1/RConn1
  Ideal Torque Source1/RConn2 -- Mechanical Rotational Reference1/LConn1

== system EcoSIM3_P2_C2/Powertrain/Electric Motor / Component Model/Sensors ==
  note: Sensor Model: Place where we add Corrupter
  Sensor In : Inport
  Bus Creator : BusCreator  Inputs=5
  Bus Selector : BusSelector  OutputSignals=InternalMotorError,EM_Temperature_degC
  Bus Selector1 : BusSelector  OutputSignals=EM_Torque_Produced_Nm,EM_Speed_produced_rad_per_s
  Fault Insertation : Subsystem
  Ideal Rotational Motion Sensor : fl_lib/Mechanical/Mechanical Sensors/Ideal Rotational Motion Sensor  offset=0 rad
  Ideal Torque Sensor : fl_lib/Mechanical/Mechanical Sensors/Ideal Torque Sensor
  Mechanical Rotational Reference1 : fl_lib/Mechanical/Rotational Elements/Mechanical Rotational Reference
  PS-Simulink Converter : nesl_utility/PS-Simulink Converter  PhysicalDomain=network_engine_domain  SubClassName=ps_output  LeftPortType=input  RightPortType=output  PseudoPeriodic=off  Frequencies=[]  Unit=1  AffineConversion=off
  PS-Simulink Converter1 : nesl_utility/PS-Simulink Converter  PhysicalDomain=network_engine_domain  SubClassName=ps_output  LeftPortType=input  RightPortType=output  PseudoPeriodic=off  Frequencies=[]  Unit=1  AffineConversion=off
  Product : Product
  Sensor lag : Subsystem
  Sensor lag1 : Subsystem
  Sensors : Subsystem
  Terminator : Terminator
  Shaft : PMIOPort  Port=1  Side=Left
  To_Plants : PMIOPort  Port=2  Side=Right
  Sensor Out : Outport
  To_Battery : Outport  Port=2
  wires:
  Bus Creator/1 -> Sensor Out/1  "EM_Sensor_Out"
  Sensor In/1 -> Bus Selector/1
  Bus Selector/1 -> Bus Creator/1  "<InternalMotorError>"
  Sensor lag/1(o) -> Terminator/1  "EM_Speed_rad_per_s"
  Sensor lag1/1(o) -> Fault Insertation/1(In1), Bus Creator/4  "EM_Torque_Out_Nm"
  Product/1 -> Bus Creator/5, To_Battery/1  "EM_Power_In_W"
  PS-Simulink Converter1/1 -> Sensor lag1/1(i)  "EM_Torque_Out_Nm"
  PS-Simulink Converter/1 -> Sensor lag/1(i)  "EM_Speed_rad_per_s"
  Sensors/1(EM_Shaft_out) -> Bus Selector1/1
  Bus Selector1/1 -> Product/1  "<EM_Torque_Produced_Nm>"
  Bus Selector1/2 -> Product/2, Bus Creator/3  "<EM_Speed_produced_rad_per_s>"
  Bus Selector/2 -> Bus Creator/2  "<EM_Temperature_degC>"
  connections:
  Shaft/RConn1 -- Ideal Rotational Motion Sensor/LConn1 -- Ideal Torque Sensor/LConn1
  Ideal Rotational Motion Sensor/RConn1 -- Mechanical Rotational Reference1/LConn1
  PS-Simulink Converter/LConn1 -- Ideal Rotational Motion Sensor/RConn2
  PS-Simulink Converter1/LConn1 -- Ideal Torque Sensor/RConn2
  Sensors/LConn1 -- Fault Insertation/RConn1 -- Ideal Torque Sensor/RConn1
  To_Plants/RConn1 -- Sensors/RConn1

== system EcoSIM3_P2_C2/Powertrain/Electric Motor /Soft ECU/Algorithm ==
  note: The batt_mainc_stat used by this model is actually the
      | bcm_mainc_stat signal transmitted by the ESS softECU
  note: Signals like T& E are used to calculate whatever is required by Soft ECU
  note: Sensor signals getting transmitted over CAN are selected here
  note: Sensor signals getting transmitted over CAN are bussed together here
  note: Signals getting transmitted to Actuators are bussed together here
  note: Feedback signals from the Normal state. Signals contain RUN_Fault and ShutdownRequest
  Inputs : Inport
  Bus Creator : BusCreator  Inputs=9
  Bus Selector : BusSelector  OutputSignals=EM_Sensors
  Bus Selector1 : BusSelector  OutputSignals=EM_Temperature_degC,Motor_Speed,EM_Torque_Out_Nm
  Bus Selector2 : BusSelector  OutputSignals=vsm_state_value,vsm_state_trigger
  Compare To Constant : simulink/Logic and Bit Operations/Compare To Constant  relop===  const=6  OutDataTypeStr=boolean
  Inverter Status : Display
  Memory : Memory
  Normal Operation : Subsystem
  Rinehart Documentation : Subsystem
      settings: OpenFcn=open('/Component_docs/RMS CAN Protocol (V4_0).pdf')
  Startup_Shutdown : Subsystem
  Switch : Switch  Criteria=u2 > Threshold  Threshold=0.5
  Temperature Values Dummy : Subsystem
  Outputs : Outport
  wires:
  Bus Selector/1 -> Bus Selector1/1, Normal Operation/4(Sensors)  "<EM_Sensors>"
  Bus Creator/1 -> Outputs/1  "EM_Out"
  Bus Selector1/2 -> Bus Creator/2  "<Motor_Speed>"
  Switch/1 -> Bus Creator/9, Compare To Constant/1  "VSM_State"
  Normal Operation/1(Commanded_Torque) -> Bus Creator/7
  Compare To Constant/1 -> Normal Operation/Enable
  Normal Operation/2(RUN_Fault) -> Bus Creator/5, Memory/1
  Inputs/1 -> Startup_Shutdown/1(SignalIn), Normal Operation/1(SignalIn), Bus Selector/1
  Memory/1 -> Startup_Shutdown/3(RUN_Fault)
  Normal Operation/3(ShutdownRequest) -> Bus Creator/4, Startup_Shutdown/4(ShutDownRequest)
  Startup_Shutdown/2(Inverter_Enable_Lockout) -> Bus Creator/6
  Startup_Shutdown/3(Inverter_Status) -> Inverter Status/1
  [GM_Transmit] -> Startup_Shutdown/2(Ignition Switch), Normal Operation/2(Ignition Switch)
  Bus Selector1/3 -> Bus Creator/3  "<EM_Torque_Out_Nm>"
  Startup_Shutdown/4(POST_Fault) -> Bus Creator/8
  Bus Selector1/1 -> Temperature Values Dummy/1(FromPlant)  "<EM_Temperature_degC>"
  Temperature Values Dummy/1(TempValues) -> Bus Creator/1  "Temperatures"
  Startup_Shutdown/1(VSM_Mode) -> Switch/3  "VSM_State"
  [VSM_State_Trigger] -> Bus Selector2/1
  Bus Selector2/2 -> Switch/2  "<vsm_state_trigger>"
  Bus Selector2/1 -> Switch/1  "<vsm_state_value>"
  [EM_Torque_Cmd_Trigger] -> Normal Operation/3(FaultTrigger)

== system EcoSIM3_P2_C2/Powertrain/Electric Motor /Soft ECU/Inputs ==
  note: Change Name according to protocol, thats what the .dbc names should be
  note: Do the input conditioning (if any) required by the
      | Algorith
  note: Select the CAN signals
  note: Select the Sensor signals
  note: Combine all the Signals that go to the
      | Soft ECU Algorithm:
      | -Calculated Signals from Sensors and CAN
      | -Signalfrom sensors pass through because they
      | need to be sent out over the CAN by the ECU
  From_ECUs : Inport
  Sensors : Inport  Port=2
  Bus Creator : BusCreator  Inputs=3
  Bus Creator1 : BusCreator
  Bus Selector : BusSelector  OutputSignals=EM_CAN_Messages,ESS_Transmit.ESS_CAN_Out
  Bus Selector1 : BusSelector  OutputSignals=EM_Temperature_degC,InternalMotorError,EM_Speed_produced_rad_per_s,EM_Torque_Out_Nm
  Gain : Gain
  To_Algorithm : Outport
  wires:
  From_ECUs/1 -> Bus Selector/1
  Sensors/1 -> Bus Selector1/1
  Bus Creator/1 -> To_Algorithm/1  "Component_to_Alg"
  Bus Selector/1 -> Bus Creator/2  "<EM_CAN_Messages>"
  Bus Selector1/3 -> Gain/1  "<EM_Speed_produced_rad_per_s>"
  Gain/1 -> Bus Creator1/3  "Motor_Speed"
  Bus Creator1/1 -> Bus Creator/1  "EM_Sensors"
  Bus Selector1/2 -> Bus Creator1/2  "<InternalMotorError>"
  Bus Selector/2 -> Bus Creator/3  "<ESS_CAN_Out>"
  Bus Selector1/4 -> Bus Creator1/4  "<EM_Torque_Out_Nm>"
  Bus Selector1/1 -> Bus Creator1/1  "<EM_Temperature_degC>"

== system EcoSIM3_P2_C2/Powertrain/Electric Motor /Soft ECU/Outputs ==
  note: Change Name according to protocol, thats what the .dbc names should be
  From Algorithm : Inport
  Bus Creator : BusCreator  Inputs=8
  Bus Creator1 : BusCreator  Inputs=1
  Bus Selector : BusSelector  OutputSignals=Temperatures,Motor_Speed,EM_Torque_Out_Nm,ShutdownRequest,RUN_Fault,Inverter_Enable_Lockout,POST_Fault,VSM_State,Commanded_Torque
  To_ECUs : Outport
  Actuator Commands : Outport  Port=2
  wires:
  Bus Creator/1 -> To_ECUs/1  "EM_Out"
  Bus Creator1/1 -> Actuator Commands/1  "EM_Actuator_Cmds"
  From Algorithm/1 -> Bus Selector/1
  Bus Selector/2 -> Bus Creator/2  "<Motor_Speed>"
  Bus Selector/4 -> Bus Creator/4  "<ShutdownRequest>"
  Bus Selector/5 -> Bus Creator/5  "<RUN_Fault>"
  Bus Selector/6 -> Bus Creator/6  "<Inverter_Enable_Lockout>"
  Bus Selector/9 -> Bus Creator1/1  "<Commanded_Torque>"
  Bus Selector/3 -> Bus Creator/3  "<EM_Torque_Out_Nm>"
  Bus Selector/7 -> Bus Creator/7  "<POST_Fault>"
  Bus Selector/8 -> Bus Creator/8  "<VSM_State>"
  Bus Selector/1 -> Bus Creator/1  "<Temperatures>"

== system EcoSIM3_P2_C2/Powertrain/Electrical Storage System/ ESS Model/Actuators ==
  note: The switch is emulating the battery contactor:
      | If the bcm_manc_stat is less than 1 there will be no power request from the ESS
  note: This is I*V Requested
  note: Actuator Model or a Signal Pass-through, Remove the bus if you are passing through all the signals
  ActuatorInputs : Inport
  Charger_P_in [W] : Inport  Port=2
  EM P_in [W] : Inport  Port=3
  Acc P_in [W] : Inport  Port=4
  BAS P_in [W] : Inport  Port=5
  Add : Sum  Inputs=++++
  Bus Creator : BusCreator  Inputs=2
  Bus Selector : BusSelector  OutputSignals=bcm_mainc_stat
  Contactors : Switch  Criteria=u2 > Threshold  Threshold=0.5
  ESS_Power_Request : Constant  Value=0
  Scope : Scope
      settings: SaveName=ScopeData3
  Actuator Outputs : Outport
  wires:
  ActuatorInputs/1 -> Bus Creator/1, Bus Selector/1
  EM P_in [W]/1 -> Add/2
  Acc P_in [W]/1 -> Add/3
  BAS P_in [W]/1 -> Add/4
  Contactors/1 -> Scope/1, Bus Creator/2  "Component_Power_Request_W"
  Bus Creator/1 -> Actuator Outputs/1  "Component_Power_Request_W"
  Bus Selector/1 -> Contactors/2  "<bcm_mainc_stat>"
  Add/1 -> Contactors/1  "Component_Power_Request_W"
  ESS_Power_Request/1 -> Contactors/3
  Charger_P_in [W]/1 -> Add/1

== system EcoSIM3_P2_C2/Powertrain/Electrical Storage System/ ESS Model/Plant ==
  note: Three kinds of Outputs:
      | 1.To_sensors: Signals that can actually be sensed through Sensors go to sensor models
      | 2. To_plants: Signals that are not actually sensed by sensors but are utilized by the rest of the plant and actually happen physically
      | Component_Logging: Logs both the signal kinds before going through sensor
  note: BATTERY MODEL
  From_Actuators : Inport
  Bus Creator : BusCreator  Inputs=5
  Bus Selector : BusSelector  OutputSignals=ESS_Actuator_Cmds.AccPwrMdlHiVltInpCrnt,Component_Power_Request_W
  Electrical Plant Model : Subsystem
  Integrator : Integrator
  Power Calculation : Subsystem
  Terminator1 : Terminator
  Terminator2 : Terminator
  Thermal Model : Subsystem
  To_Sensors : Outport
  wires:
  Bus Creator/1 -> To_Sensors/1  "ESS_to_sensors"
  From_Actuators/1 -> Bus Selector/1
  Electrical Plant Model/1(Batt_Current [A]) -> Integrator/1, Bus Creator/2
  Electrical Plant Model/2(Batt_SOC [%]) -> Bus Creator/3
  Electrical Plant Model/3(Batt_volt [V]) -> Bus Creator/4
  Thermal Model/1(Batt_Temp [C]) -> Electrical Plant Model/2(Batt_Temp [C]), Bus Creator/5
  Bus Selector/1 -> Power Calculation/1(Input_Crnt [A])  "<AccPwrMdlHiVltInpCrnt>"
  Power Calculation/1(P_in [W]) -> Electrical Plant Model/1(P_in [W])
  Electrical Plant Model/5(Batt_volt_1 [V]) -> Power Calculation/2(Batt_volt_1 [V])
  Electrical Plant Model/4(Batt_Heat [W]) -> Thermal Model/1(Batt_Heat [W])
  Integrator/1 -> Bus Creator/1  "BATT_cap_used"
  Power Calculation/2(Batt_Electrical_Energy) -> Terminator1/1
  Power Calculation/3(Batt_Electrical_Energy_Net) -> Terminator2/1
  Bus Selector/2 -> Power Calculation/3(Component_Power_Watts)  "<Component_Power_Request_W>"

== system EcoSIM3_P2_C2/Powertrain/Electrical Storage System/ ESS Model/Sensors ==
  note: Sensor Model: Place where we add Corrupter
  Sensor In : Inport
  Bus Creator : BusCreator
  Bus Selector : BusSelector  OutputSignals=Batt_Current_A,Batt_SOC_percent,Batt_Temp_C,Batt_Voltage_V
  Sensor Out : Outport
  wires:
  Bus Creator/1 -> Sensor Out/1  "ESS_Sensor_Out"
  Sensor In/1 -> Bus Selector/1
  Bus Selector/1 -> Bus Creator/1  "<Batt_Current_A>"
  Bus Selector/2 -> Bus Creator/2  "<Batt_SOC_percent>"
  Bus Selector/3 -> Bus Creator/3  "<Batt_Temp_C>"
  Bus Selector/4 -> Bus Creator/4  "<Batt_Voltage_V>"

== system EcoSIM3_P2_C2/Powertrain/Electrical Storage System/Soft ECU/Algorithm ==
  note: Signals like T& E are used to calculate whatever is required by Soft ECU
  note: Sensor signals getting transmitted over CAN are selected here
  note: Sensor signals getting transmitted over CAN are bussed together here
  note: Sensor signals getting transmitted over CAN are selected here
  Inputs : Inport
  A123 Documentation : Subsystem
      settings: OpenFcn=open('/Component_docs/EcoCAR A123 ICD v1.pdf')
  A123 soft ECU : Subsystem
  Bus Creator1 : BusCreator  Inputs=9
  Bus Creator2 : BusCreator  Inputs=8
  Bus Selector : BusSelector  OutputSignals=AccPwrMdlHiVltInpCrnt,Component_Sensor_Out,hsc_bcm_enable,hsc_bcm_mainc_close,hsc_bcm_leakage_ena,hsc_bcm_epo,BMS_Powerup,chga_wake,Component_Sensor_Out.Batt_Temp_C
  Bus Selector1 : BusSelector  OutputSignals=Batt_SOC_percent,Batt_Voltage_V,Batt_Current_A
  Bus Selector2 : BusSelector  OutputSignals=bcm_mainc_stat
  Gain : Gain  Gain=1.1
  Gain1 : Gain  Gain=0.8
  Outputs : Outport
  wires:
  Inputs/1 -> Bus Selector/1
  Bus Creator1/1 -> Outputs/1  "ESS_SoftECU_Out"
  Bus Selector1/1 -> Bus Creator1/4  "<Batt_SOC_percent>"
  Bus Selector/1 -> Bus Creator1/1  "<AccPwrMdlHiVltInpCrnt>"
  Bus Creator2/1 -> A123 soft ECU/1(From ECUs)
  Gain1/1 -> Bus Creator1/9, Bus Creator2/5  "bcm_cell_tmin"
  Gain/1 -> Bus Creator1/8, Bus Creator2/4  "bcm_cell_tmax"
  Bus Selector/2 -> Bus Selector1/1  "<Component_Sensor_Out>"
  Bus Selector/4 -> Bus Creator2/2, Bus Creator1/2  "<hsc_bcm_mainc_close>"
  A123 soft ECU/1(To ECUs) -> Bus Creator1/5, Bus Selector2/1  "SoftECU_Out"
  Bus Selector/3 -> Bus Creator2/1  "<hsc_bcm_enable>"
  Bus Selector2/1 -> Bus Creator1/3  "<bcm_mainc_stat>"
  Bus Selector/5 -> Bus Creator2/3  "<hsc_bcm_leakage_ena>"
  Bus Selector1/2 -> Bus Creator1/6  "<Batt_Voltage_V>"
  Bus Selector1/3 -> Bus Creator1/7  "<Batt_Current_A>"
  Bus Selector/6 -> Bus Creator2/6  "<hsc_bcm_epo>"
  Bus Selector/7 -> Bus Creator2/7  "<BMS_Powerup>"
  Bus Selector/8 -> Bus Creator2/8  "<chga_wake>"
  Bus Selector/9 -> Gain1/1, Gain/1  "<Batt_Temp_C>"

== system EcoSIM3_P2_C2/Powertrain/Electrical Storage System/Soft ECU/Inputs ==
  note: Do the input conditioning (if any) required by the
      | Algorith
  note: Select the CAN signals
  note: Select the Sensor signals
  note: Combine all the Signals that go to the
      | Soft ECU Algorithm:
      | -Calculated Signals from Sensors and CAN
      | -Signalfrom sensors pass through because they
      | need to be sent out over the CAN by the ECU
  Sensors : Inport
  CAN_In : Inport  Port=2
  Bus Creator : BusCreator  Inputs=8
  Bus Selector : BusSelector  OutputSignals=AccPwrMdlHiVltInpCrnt,hsc_bcm_mainc_close,hsc_bcm_enable,hsc_bcm_leakage_ena,hsc_bcm_epo,BMS_Powerup,chga_wake
  To_Algorithm : Outport
  wires:
  CAN_In/1 -> Bus Selector/1
  Sensors/1 -> Bus Creator/1
  Bus Creator/1 -> To_Algorithm/1  "Component_to_Alg"
  Bus Selector/1 -> Bus Creator/2  "<AccPwrMdlHiVltInpCrnt>"
  Bus Selector/2 -> Bus Creator/3  "<hsc_bcm_mainc_close>"
  Bus Selector/3 -> Bus Creator/4  "<hsc_bcm_enable>"
  Bus Selector/4 -> Bus Creator/5  "<hsc_bcm_leakage_ena>"
  Bus Selector/5 -> Bus Creator/6  "<hsc_bcm_epo>"
  Bus Selector/6 -> Bus Creator/7  "<BMS_Powerup>"
  Bus Selector/7 -> Bus Creator/8  "<chga_wake>"

== system EcoSIM3_P2_C2/Powertrain/Electrical Storage System/Soft ECU/Outputs ==
  note: Select the Sensor signals
  From Algorithm : Inport
  Bus Creator2 : BusCreator  Inputs=6
  Bus Creator3 : BusCreator  Inputs=2
  Bus Selector : BusSelector  OutputSignals=AccPwrMdlHiVltInpCrnt,bcm_mainc_stat,Batt_SOC_percent,SoftECU_Out,Batt_Voltage_V,Batt_Current_A,bcm_cell_tmax,bcm_cell_tmin
  Actuator_Cmds : Outport
  To ECUs : Outport  Port=2
  wires:
  Bus Selector/4 -> Bus Creator2/2  "<SoftECU_Out>"
  Bus Selector/3 -> Bus Creator2/1  "<Batt_SOC_percent>"
  Bus Selector/2 -> Bus Creator3/2  "<bcm_mainc_stat>"
  Bus Selector/1 -> Bus Creator3/1  "<AccPwrMdlHiVltInpCrnt>"
  From Algorithm/1 -> Bus Selector/1
  Bus Creator2/1 -> To ECUs/1  "ESS_CAN_Out"
  Bus Creator3/1 -> Actuator_Cmds/1  "ESS_Actuator_Cmds"
  Bus Selector/5 -> Bus Creator2/3  "<Batt_Voltage_V>"
  Bus Selector/6 -> Bus Creator2/4  "<Batt_Current_A>"
  Bus Selector/7 -> Bus Creator2/5  "<bcm_cell_tmax>"
  Bus Selector/8 -> Bus Creator2/6  "<bcm_cell_tmin>"

== system EcoSIM3_P2_C2/Powertrain/Engine/ Component Model/Actuators ==
  note: Actuator Model or a Signal Pass-through, Remove the bus if you are passing through all the signals
  ActuatorInputs : Inport
  Actuator Outputs : Outport
  wires:
  ActuatorInputs/1 -> Actuator Outputs/1
